simulink model "UserVehicle_RTW"  (Simulink 7.5)
settings: Solver=ode1  SolverMode=SingleTasking  StartTime=0.0  StopTime=inf  FixedStep=0.001  RelTol=1e-3
PreLoadFcn:
  | vehicle = 'Car'; if ~length(which('cmcmd')), cmenv; end
  | UserVehicle_RTW_bus
  | UserVehicle_RTW_params
InitFcn:
  | vehicle = 'Car'; if ~length(which('cmcmd')), cmenv; end
  | UserVehicle_RTW_bus
  | UserVehicle_RTW_params
values from neighbouring files (symbols this model uses):
  Car_Bdy1_mass = 650.0    (= 650)    [SingleTrack_RTW_params.m]    (also in UserVehicle_RTW_params.m)
  Car_Steering_i = 10.0    (= 10)    [SingleTrack_RTW_params.m]    (also in UserVehicle_RTW_params.m)
  Car_WhlBaseF = 1.5    [SingleTrack_RTW_params.m]    (also in UserVehicle_RTW_params.m)
  Car_WhlBaseR = -1.5    [SingleTrack_RTW_params.m]    (also in UserVehicle_RTW_params.m)
libraries: CarMaker4SL x77
(part 2 of 3)

== system UserVehicle_RTW/SingleTrack_Out/Subsystem1 ==
  In1 : Inport  OutDataType=sfix(16)  OutScaling=2^0
  Bus Creator : BusCreator  Inputs=3
  foo_Input_Selector1 : BusSelector  OutputSignals=Vhcl v,Vhcl Distance,Vhcl sRoad,Vhcl sRoadAero,Vhcl Hitch_Pos x,Vhcl Hitch_Pos y,Vhcl Hitch_Pos z,Vhcl Roll,Vhcl RollVel,Vhcl RollAcc,Vhcl Pitch,Vhcl PitchVel,Vhcl PitchAcc,Vhcl Yaw,Vhcl YawRate,Vhcl YawAcc
  Out1 : Outport  OutDataType=sfix(16)  OutScaling=2^0
  Out2 : Outport  Port=2  OutDataType=sfix(16)  OutScaling=2^0
  Out3 : Outport  Port=3  OutDataType=sfix(16)  OutScaling=2^0
  Out4 : Outport  Port=4  OutDataType=sfix(16)  OutScaling=2^0
  Out6 : Outport  Port=5  OutDataType=sfix(16)  OutScaling=2^0
  Out7 : Outport  Port=6  OutDataType=sfix(16)  OutScaling=2^0
  Out8 : Outport  Port=7  OutDataType=sfix(16)  OutScaling=2^0
  Out9 : Outport  Port=8  OutDataType=sfix(16)  OutScaling=2^0
  Out10 : Outport  Port=9  OutDataType=sfix(16)  OutScaling=2^0
  Out11 : Outport  Port=10  OutDataType=sfix(16)  OutScaling=2^0
  Out12 : Outport  Port=11  OutDataType=sfix(16)  OutScaling=2^0
  Out13 : Outport  Port=12  OutDataType=sfix(16)  OutScaling=2^0
  Out14 : Outport  Port=13  OutDataType=sfix(16)  OutScaling=2^0
  Out15 : Outport  Port=14  OutDataType=sfix(16)  OutScaling=2^0
  wires:
  In1/1 -> foo_Input_Selector1/1
  foo_Input_Selector1/16 -> Out15/1  "<Vhcl YawAcc>"
  foo_Input_Selector1/15 -> Out14/1  "<Vhcl YawRate>"
  foo_Input_Selector1/14 -> Out13/1  "<Vhcl Yaw>"
  foo_Input_Selector1/13 -> Out12/1  "<Vhcl PitchAcc>"
  foo_Input_Selector1/12 -> Out11/1  "<Vhcl PitchVel>"
  foo_Input_Selector1/11 -> Out10/1  "<Vhcl Pitch>"
  foo_Input_Selector1/10 -> Out9/1  "<Vhcl RollAcc>"
  foo_Input_Selector1/9 -> Out8/1  "<Vhcl RollVel>"
  foo_Input_Selector1/8 -> Out7/1  "<Vhcl Roll>"
  Bus Creator/1 -> Out6/1
  foo_Input_Selector1/4 -> Out4/1  "<Vhcl sRoadAero>"
  foo_Input_Selector1/3 -> Out3/1  "<Vhcl sRoad>"
  foo_Input_Selector1/2 -> Out2/1  "<Vhcl Distance>"
  foo_Input_Selector1/1 -> Out1/1  "<Vhcl v>"
  foo_Input_Selector1/7 -> Bus Creator/3  "<Vhcl Hitch_Pos z>"
  foo_Input_Selector1/6 -> Bus Creator/2  "<Vhcl Hitch_Pos y>"
  foo_Input_Selector1/5 -> Bus Creator/1  "<Vhcl Hitch_Pos x>"

== system UserVehicle_RTW/SingleTrack_Out/Subsystem2 ==
  In1 : Inport  OutDataType=sfix(16)  OutScaling=2^0
  Bus Creator : BusCreator  Inputs=3
  Bus Creator1 : BusCreator  Inputs=3
  foo_Input_Selector3 : BusSelector  OutputSignals=Vhcl Wheel FL t x,Vhcl Wheel FL t y,Vhcl Wheel FL t z,Vhcl Wheel FL r_zxy x,Vhcl Wheel FL r_zxy y,Vhcl Wheel FL r_zxy z,Vhcl Wheel FL Fx,Vhcl Wheel FL Fy,Vhcl Wheel FL Fz,Vhcl Wheel FL vBelt,Vhcl Wheel FL LongSlip,Vhcl Wheel FL SideSlip,Vhcl Wheel FL Trq_T2W,Vhcl Wheel FL Trq_WhlBearing
  Out1 : Outport  OutDataType=sfix(16)  OutScaling=2^0
  Out2 : Outport  Port=2  OutDataType=sfix(16)  OutScaling=2^0
  Out3 : Outport  Port=3  OutDataType=sfix(16)  OutScaling=2^0
  Out4 : Outport  Port=4  OutDataType=sfix(16)  OutScaling=2^0
  Out5 : Outport  Port=5  OutDataType=sfix(16)  OutScaling=2^0
  Out6 : Outport  Port=6  OutDataType=sfix(16)  OutScaling=2^0
  Out7 : Outport  Port=7  OutDataType=sfix(16)  OutScaling=2^0
  Out8 : Outport  Port=8  OutDataType=sfix(16)  OutScaling=2^0
  Out9 : Outport  Port=9  OutDataType=sfix(16)  OutScaling=2^0
  Out10 : Outport  Port=10  OutDataType=sfix(16)  OutScaling=2^0
  wires:
  foo_Input_Selector3/14 -> Out10/1  "<Vhcl Wheel FL Trq_WhlBearing>"
  foo_Input_Selector3/13 -> Out9/1  "<Vhcl Wheel FL Trq_T2W>"
  foo_Input_Selector3/12 -> Out8/1  "<Vhcl Wheel FL SideSlip>"
  foo_Input_Selector3/11 -> Out7/1  "<Vhcl Wheel FL LongSlip>"
  foo_Input_Selector3/10 -> Out6/1  "<Vhcl Wheel FL vBelt>"
  foo_Input_Selector3/9 -> Out5/1  "<Vhcl Wheel FL Fz>"
  foo_Input_Selector3/8 -> Out4/1  "<Vhcl Wheel FL Fy>"
  In1/1 -> foo_Input_Selector3/1
  foo_Input_Selector3/7 -> Out3/1  "<Vhcl Wheel FL Fx>"
  Bus Creator/1 -> Out2/1
  Bus Creator1/1 -> Out1/1
  foo_Input_Selector3/6 -> Bus Creator/3  "<Vhcl Wheel FL r_zxy z>"
  foo_Input_Selector3/5 -> Bus Creator/2  "<Vhcl Wheel FL r_zxy y>"
  foo_Input_Selector3/4 -> Bus Creator/1  "<Vhcl Wheel FL r_zxy x>"
  foo_Input_Selector3/3 -> Bus Creator1/3  "<Vhcl Wheel FL t z>"
  foo_Input_Selector3/2 -> Bus Creator1/2  "<Vhcl Wheel FL t y>"
  foo_Input_Selector3/1 -> Bus Creator1/1  "<Vhcl Wheel FL t x>"

== system UserVehicle_RTW/SingleTrack_Out/Subsystem3 ==
  In1 : Inport  OutDataType=sfix(16)  OutScaling=2^0
  Bus Creator : BusCreator  Inputs=3
  Bus Creator1 : BusCreator  Inputs=3
  foo_Input_Selector3 : BusSelector  OutputSignals=Vhcl Wheel FR t x,Vhcl Wheel FR t y,Vhcl Wheel FR t z,Vhcl Wheel FR r_zxy x,Vhcl Wheel FR r_zxy y,Vhcl Wheel FR r_zxy z,Vhcl Wheel FR Fx,Vhcl Wheel FR Fy,Vhcl Wheel FR Fz,Vhcl Wheel FR vBelt,Vhcl Wheel FR LongSlip,Vhcl Wheel FR SideSlip,Vhcl Wheel FR Trq_T2W,Vhcl Wheel FR Trq_WhlBearing
  Out1 : Outport  OutDataType=sfix(16)  OutScaling=2^0
  Out2 : Outport  Port=2  OutDataType=sfix(16)  OutScaling=2^0
  Out3 : Outport  Port=3  OutDataType=sfix(16)  OutScaling=2^0
  Out4 : Outport  Port=4  OutDataType=sfix(16)  OutScaling=2^0
  Out5 : Outport  Port=5  OutDataType=sfix(16)  OutScaling=2^0
  Out6 : Outport  Port=6  OutDataType=sfix(16)  OutScaling=2^0
  Out7 : Outport  Port=7  OutDataType=sfix(16)  OutScaling=2^0
  Out8 : Outport  Port=8  OutDataType=sfix(16)  OutScaling=2^0
  Out9 : Outport  Port=9  OutDataType=sfix(16)  OutScaling=2^0
  Out10 : Outport  Port=10  OutDataType=sfix(16)  OutScaling=2^0
  wires:
  foo_Input_Selector3/14 -> Out10/1  "<Vhcl Wheel FR Trq_WhlBearing>"
  foo_Input_Selector3/13 -> Out9/1  "<Vhcl Wheel FR Trq_T2W>"
  foo_Input_Selector3/12 -> Out8/1  "<Vhcl Wheel FR SideSlip>"
  foo_Input_Selector3/11 -> Out7/1  "<Vhcl Wheel FR LongSlip>"
  foo_Input_Selector3/10 -> Out6/1  "<Vhcl Wheel FR vBelt>"
  foo_Input_Selector3/9 -> Out5/1  "<Vhcl Wheel FR Fz>"
  foo_Input_Selector3/8 -> Out4/1  "<Vhcl Wheel FR Fy>"
  In1/1 -> foo_Input_Selector3/1
  foo_Input_Selector3/7 -> Out3/1  "<Vhcl Wheel FR Fx>"
  Bus Creator1/1 -> Out2/1
  Bus Creator/1 -> Out1/1
  foo_Input_Selector3/6 -> Bus Creator1/3  "<Vhcl Wheel FR r_zxy z>"
  foo_Input_Selector3/5 -> Bus Creator1/2  "<Vhcl Wheel FR r_zxy y>"
  foo_Input_Selector3/4 -> Bus Creator1/1  "<Vhcl Wheel FR r_zxy x>"
  foo_Input_Selector3/3 -> Bus Creator/3  "<Vhcl Wheel FR t z>"
  foo_Input_Selector3/2 -> Bus Creator/2  "<Vhcl Wheel FR t y>"
  foo_Input_Selector3/1 -> Bus Creator/1  "<Vhcl Wheel FR t x>"

== system UserVehicle_RTW/SingleTrack_Out/Subsystem4 ==
  In1 : Inport  OutDataType=sfix(16)  OutScaling=2^0
  Bus Creator : BusCreator  Inputs=3
  Bus Creator1 : BusCreator  Inputs=3
  foo_Input_Selector3 : BusSelector  OutputSignals=Vhcl Wheel RL t x,Vhcl Wheel RL t y,Vhcl Wheel RL t z,Vhcl Wheel RL r_zxy x,Vhcl Wheel RL r_zxy y,Vhcl Wheel RL r_zxy z,Vhcl Wheel RL Fx,Vhcl Wheel RL Fy,Vhcl Wheel RL Fz,Vhcl Wheel RL vBelt,Vhcl Wheel RL LongSlip,Vhcl Wheel RL SideSlip,Vhcl Wheel RL Trq_T2W,Vhcl Wheel RL Trq_WhlBearing
  Out1 : Outport  OutDataType=sfix(16)  OutScaling=2^0
  Out2 : Outport  Port=2  OutDataType=sfix(16)  OutScaling=2^0
  Out3 : Outport  Port=3  OutDataType=sfix(16)  OutScaling=2^0
  Out4 : Outport  Port=4  OutDataType=sfix(16)  OutScaling=2^0
  Out5 : Outport  Port=5  OutDataType=sfix(16)  OutScaling=2^0
  Out6 : Outport  Port=6  OutDataType=sfix(16)  OutScaling=2^0
  Out7 : Outport  Port=7  OutDataType=sfix(16)  OutScaling=2^0
  Out8 : Outport  Port=8  OutDataType=sfix(16)  OutScaling=2^0
  Out9 : Outport  Port=9  OutDataType=sfix(16)  OutScaling=2^0
  Out10 : Outport  Port=10  OutDataType=sfix(16)  OutScaling=2^0
  wires:
  foo_Input_Selector3/14 -> Out10/1  "<Vhcl Wheel RL Trq_WhlBearing>"
  foo_Input_Selector3/13 -> Out9/1  "<Vhcl Wheel RL Trq_T2W>"
  foo_Input_Selector3/12 -> Out8/1  "<Vhcl Wheel RL SideSlip>"
  foo_Input_Selector3/11 -> Out7/1  "<Vhcl Wheel RL LongSlip>"
  foo_Input_Selector3/10 -> Out6/1  "<Vhcl Wheel RL vBelt>"
  foo_Input_Selector3/9 -> Out5/1  "<Vhcl Wheel RL Fz>"
  foo_Input_Selector3/8 -> Out4/1  "<Vhcl Wheel RL Fy>"
  In1/1 -> foo_Input_Selector3/1
  foo_Input_Selector3/7 -> Out3/1  "<Vhcl Wheel RL Fx>"
  Bus Creator1/1 -> Out2/1
  Bus Creator/1 -> Out1/1
  foo_Input_Selector3/6 -> Bus Creator1/3  "<Vhcl Wheel RL r_zxy z>"
  foo_Input_Selector3/5 -> Bus Creator1/2  "<Vhcl Wheel RL r_zxy y>"
  foo_Input_Selector3/4 -> Bus Creator1/1  "<Vhcl Wheel RL r_zxy x>"
  foo_Input_Selector3/3 -> Bus Creator/3  "<Vhcl Wheel RL t z>"
  foo_Input_Selector3/2 -> Bus Creator/2  "<Vhcl Wheel RL t y>"
  foo_Input_Selector3/1 -> Bus Creator/1  "<Vhcl Wheel RL t x>"

== system UserVehicle_RTW/SingleTrack_Out/Subsystem5 ==
  In1 : Inport  OutDataType=sfix(16)  OutScaling=2^0
  Bus Creator : BusCreator  Inputs=3
  Bus Creator1 : BusCreator  Inputs=3
  foo_Input_Selector3 : BusSelector  OutputSignals=Vhcl Wheel RR t x,Vhcl Wheel RR t y,Vhcl Wheel RR t z,Vhcl Wheel RR r_zxy x,Vhcl Wheel RR r_zxy y,Vhcl Wheel RR r_zxy z,Vhcl Wheel RR Fx,Vhcl Wheel RR Fy,Vhcl Wheel RR Fz,Vhcl Wheel RR vBelt,Vhcl Wheel RR LongSlip,Vhcl Wheel RR SideSlip,Vhcl Wheel RR Trq_T2W,Vhcl Wheel RR Trq_WhlBearing
  Out1 : Outport  OutDataType=sfix(16)  OutScaling=2^0
  Out2 : Outport  Port=2  OutDataType=sfix(16)  OutScaling=2^0
  Out3 : Outport  Port=3  OutDataType=sfix(16)  OutScaling=2^0
  Out4 : Outport  Port=4  OutDataType=sfix(16)  OutScaling=2^0
  Out5 : Outport  Port=5  OutDataType=sfix(16)  OutScaling=2^0
  Out6 : Outport  Port=6  OutDataType=sfix(16)  OutScaling=2^0
  Out7 : Outport  Port=7  OutDataType=sfix(16)  OutScaling=2^0
  Out8 : Outport  Port=8  OutDataType=sfix(16)  OutScaling=2^0
  Out9 : Outport  Port=9  OutDataType=sfix(16)  OutScaling=2^0
  Out10 : Outport  Port=10  OutDataType=sfix(16)  OutScaling=2^0
  wires:
  foo_Input_Selector3/14 -> Out10/1  "<Vhcl Wheel RR Trq_WhlBearing>"
  foo_Input_Selector3/13 -> Out9/1  "<Vhcl Wheel RR Trq_T2W>"
  foo_Input_Selector3/12 -> Out8/1  "<Vhcl Wheel RR SideSlip>"
  foo_Input_Selector3/11 -> Out7/1  "<Vhcl Wheel RR LongSlip>"
  foo_Input_Selector3/10 -> Out6/1  "<Vhcl Wheel RR vBelt>"
  foo_Input_Selector3/9 -> Out5/1  "<Vhcl Wheel RR Fz>"
  foo_Input_Selector3/8 -> Out4/1  "<Vhcl Wheel RR Fy>"
  In1/1 -> foo_Input_Selector3/1
  foo_Input_Selector3/7 -> Out3/1  "<Vhcl Wheel RR Fx>"
  Bus Creator1/1 -> Out2/1
  Bus Creator/1 -> Out1/1
  foo_Input_Selector3/6 -> Bus Creator1/3  "<Vhcl Wheel RR r_zxy z>"
  foo_Input_Selector3/5 -> Bus Creator1/2  "<Vhcl Wheel RR r_zxy y>"
  foo_Input_Selector3/4 -> Bus Creator1/1  "<Vhcl Wheel RR r_zxy x>"
  foo_Input_Selector3/3 -> Bus Creator/3  "<Vhcl Wheel RR t z>"
  foo_Input_Selector3/2 -> Bus Creator/2  "<Vhcl Wheel RR t y>"
  foo_Input_Selector3/1 -> Bus Creator/1  "<Vhcl Wheel RR t x>"

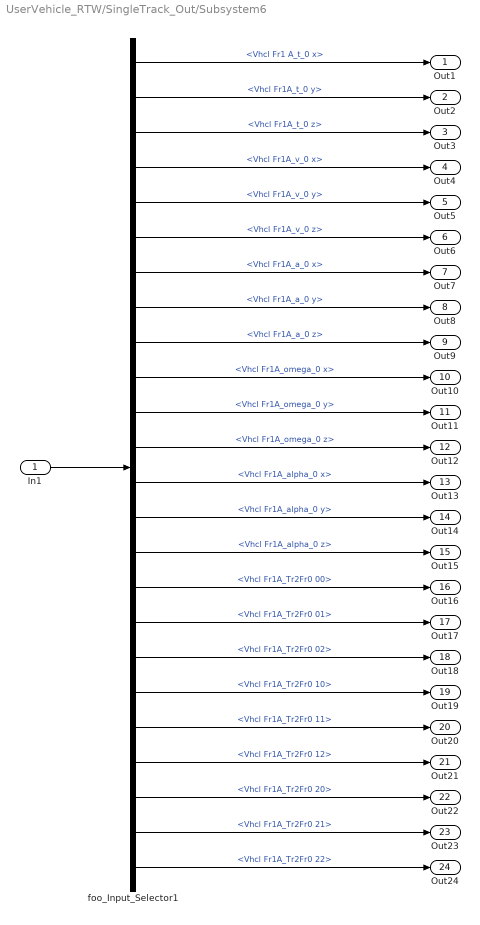
== system UserVehicle_RTW/SingleTrack_Out/Subsystem6 ==
  In1 : Inport  OutDataType=sfix(16)  OutScaling=2^0
  foo_Input_Selector1 : BusSelector  OutputSignals=Vhcl Fr1 A_t_0 x,Vhcl Fr1A_t_0 y,Vhcl Fr1A_t_0 z,Vhcl Fr1A_v_0 x,Vhcl Fr1A_v_0 y,Vhcl Fr1A_v_0 z,Vhcl Fr1A_a_0 x,Vhcl Fr1A_a_0 y,Vhcl Fr1A_a_0 z,Vhcl Fr1A_omega_0 x,Vhcl Fr1A_omega_0 y,Vhcl Fr1A_omega_0 z,Vhcl Fr1A_alpha_0 x,Vhcl Fr1A_alpha_0 y,Vhcl Fr1A_alpha_0 z,Vhcl Fr1A_Tr2Fr0 00,Vhcl Fr1A_Tr2Fr0 01,Vhcl Fr1A_Tr2Fr0 02,Vhcl Fr1A_Tr2Fr0 10,Vhcl Fr1A_Tr2Fr0 11,Vhcl Fr1A_Tr2Fr0 12,Vhcl Fr1A_Tr2Fr0 20,Vhcl Fr1A_Tr2Fr0 21,Vhcl Fr1A_Tr2Fr0 22
  Out1 : Outport  OutDataType=sfix(16)  OutScaling=2^0
  Out2 : Outport  Port=2  OutDataType=sfix(16)  OutScaling=2^0
  Out3 : Outport  Port=3  OutDataType=sfix(16)  OutScaling=2^0
  Out4 : Outport  Port=4  OutDataType=sfix(16)  OutScaling=2^0
  Out5 : Outport  Port=5  OutDataType=sfix(16)  OutScaling=2^0
  Out6 : Outport  Port=6  OutDataType=sfix(16)  OutScaling=2^0
  Out7 : Outport  Port=7  OutDataType=sfix(16)  OutScaling=2^0
  Out8 : Outport  Port=8  OutDataType=sfix(16)  OutScaling=2^0
  Out9 : Outport  Port=9  OutDataType=sfix(16)  OutScaling=2^0
  Out10 : Outport  Port=10  OutDataType=sfix(16)  OutScaling=2^0
  Out11 : Outport  Port=11  OutDataType=sfix(16)  OutScaling=2^0
  Out12 : Outport  Port=12  OutDataType=sfix(16)  OutScaling=2^0
  Out13 : Outport  Port=13  OutDataType=sfix(16)  OutScaling=2^0
  Out14 : Outport  Port=14  OutDataType=sfix(16)  OutScaling=2^0
  Out15 : Outport  Port=15  OutDataType=sfix(16)  OutScaling=2^0
  Out16 : Outport  Port=16  OutDataType=sfix(16)  OutScaling=2^0
  Out17 : Outport  Port=17  OutDataType=sfix(16)  OutScaling=2^0
  Out18 : Outport  Port=18  OutDataType=sfix(16)  OutScaling=2^0
  Out19 : Outport  Port=19  OutDataType=sfix(16)  OutScaling=2^0
  Out20 : Outport  Port=20  OutDataType=sfix(16)  OutScaling=2^0
  Out21 : Outport  Port=21  OutDataType=sfix(16)  OutScaling=2^0
  Out22 : Outport  Port=22  OutDataType=sfix(16)  OutScaling=2^0
  Out23 : Outport  Port=23  OutDataType=sfix(16)  OutScaling=2^0
  Out24 : Outport  Port=24  OutDataType=sfix(16)  OutScaling=2^0
  wires:
  foo_Input_Selector1/15 -> Out15/1  "<Vhcl Fr1A_alpha_0 z>"
  foo_Input_Selector1/14 -> Out14/1  "<Vhcl Fr1A_alpha_0 y>"
  foo_Input_Selector1/13 -> Out13/1  "<Vhcl Fr1A_alpha_0 x>"
  foo_Input_Selector1/12 -> Out12/1  "<Vhcl Fr1A_omega_0 z>"
  foo_Input_Selector1/11 -> Out11/1  "<Vhcl Fr1A_omega_0 y>"
  foo_Input_Selector1/10 -> Out10/1  "<Vhcl Fr1A_omega_0 x>"
  foo_Input_Selector1/9 -> Out9/1  "<Vhcl Fr1A_a_0 z>"
  foo_Input_Selector1/8 -> Out8/1  "<Vhcl Fr1A_a_0 y>"
  foo_Input_Selector1/7 -> Out7/1  "<Vhcl Fr1A_a_0 x>"
  foo_Input_Selector1/6 -> Out6/1  "<Vhcl Fr1A_v_0 z>"
  foo_Input_Selector1/5 -> Out5/1  "<Vhcl Fr1A_v_0 y>"
  foo_Input_Selector1/4 -> Out4/1  "<Vhcl Fr1A_v_0 x>"
  foo_Input_Selector1/3 -> Out3/1  "<Vhcl Fr1A_t_0 z>"
  foo_Input_Selector1/2 -> Out2/1  "<Vhcl Fr1A_t_0 y>"
  foo_Input_Selector1/1 -> Out1/1  "<Vhcl Fr1 A_t_0 x>"
  In1/1 -> foo_Input_Selector1/1
  foo_Input_Selector1/16 -> Out16/1  "<Vhcl Fr1A_Tr2Fr0 00>"
  foo_Input_Selector1/17 -> Out17/1  "<Vhcl Fr1A_Tr2Fr0 01>"
  foo_Input_Selector1/18 -> Out18/1  "<Vhcl Fr1A_Tr2Fr0 02>"
  foo_Input_Selector1/19 -> Out19/1  "<Vhcl Fr1A_Tr2Fr0 10>"
  foo_Input_Selector1/20 -> Out20/1  "<Vhcl Fr1A_Tr2Fr0 11>"
  foo_Input_Selector1/21 -> Out21/1  "<Vhcl Fr1A_Tr2Fr0 12>"
  foo_Input_Selector1/22 -> Out22/1  "<Vhcl Fr1A_Tr2Fr0 20>"
  foo_Input_Selector1/23 -> Out23/1  "<Vhcl Fr1A_Tr2Fr0 21>"
  foo_Input_Selector1/24 -> Out24/1  "<Vhcl Fr1A_Tr2Fr0 22>"

== system UserVehicle_RTW/UserVehicle/CreateBus Car.Hitch.FrcTrq ==
  Bus Creator : BusCreator  Inputs=6
  Constant{1..2,7..10} (6 alike) : Constant  Value=0
  Demux7 : Demux  Outputs=6
  Mux1 : Mux  Inputs=6
  Car.Hitch.FrcTrq : Outport
  wires:
  Constant1/1 -> Mux1/6
  Constant2/1 -> Mux1/5
  Constant7/1 -> Mux1/1
  Constant10/1 -> Mux1/4
  Constant9/1 -> Mux1/3
  Constant8/1 -> Mux1/2
  Mux1/1 -> Demux7/1
  Bus Creator/1 -> Car.Hitch.FrcTrq/1
  Demux7/6 -> Bus Creator/6  "Car Hitch Trq2Car z"
  Demux7/5 -> Bus Creator/5  "Car Hitch Trq2Car y"
  Demux7/4 -> Bus Creator/4  "Car Hitch Trq2Car x"
  Demux7/3 -> Bus Creator/3  "Car Hitch Frc2Car z"
  Demux7/2 -> Bus Creator/2  "Car Hitch Frc2Car y"
  Demux7/1 -> Bus Creator/1  "Car Hitch Frc2Car x"

== system UserVehicle_RTW/UserVehicle/CreateBus Vhcl.Fr1 ==
  Vhcl.Fr1_In : Inport
  BdyFrame2Vhcl.Fr1A : Subsystem
  Ground : Ground
  Ground1 : Ground
  Tr2Fr0 : Subsystem
  a_0 : Subsystem
  t_0 : Subsystem
  v_0 : Subsystem
  Vhcl.Fr1A : Outport
  wires:
  Ground/1 -> BdyFrame2Vhcl.Fr1A/5(alpha_0)
  Ground1/1 -> BdyFrame2Vhcl.Fr1A/4(omega_0)
  a_0/1(a_0) -> BdyFrame2Vhcl.Fr1A/3(a_0)
  v_0/1(v_0) -> BdyFrame2Vhcl.Fr1A/2(v_0)
  t_0/1(t_0) -> BdyFrame2Vhcl.Fr1A/1(t_0)
  Tr2Fr0/1(Tr2Fr0) -> BdyFrame2Vhcl.Fr1A/6(Tr2Fr0), a_0/2(Tr2Fr0), v_0/2(Tr2Fr0)
  Vhcl.Fr1_In/1 -> Tr2Fr0/1(Car), t_0/1(Car), v_0/1(Car), a_0/1(Car)
  BdyFrame2Vhcl.Fr1A/1(Vhcl.Fr1) -> Vhcl.Fr1A/1

== system UserVehicle_RTW/UserVehicle/CreateBus Vhcl.Misc ==
  In1 : Inport
  Bus Creator5 : BusCreator  Inputs=11
  Demux5 : Demux  Outputs=11
  Out1 : Outport
  wires:
  Demux5/11 -> Bus Creator5/11  "Vhcl Wind_vel_0 z"
  Demux5/10 -> Bus Creator5/10  "Vhcl Wind_vel_0 y"
  Demux5/9 -> Bus Creator5/9  "Vhcl Wind_vel_0 x"
  Demux5/8 -> Bus Creator5/8  "Vhcl DL2BdyEng y"
  Demux5/7 -> Bus Creator5/7  "Vhcl DL2BdyEng x"
  Demux5/6 -> Bus Creator5/6  "Vhcl TrqDL2Bdy1B z"
  Demux5/5 -> Bus Creator5/5  "Vhcl TrqDL2Bdy1B y"
  Demux5/4 -> Bus Creator5/4  "Vhcl TrqDL2Bdy1B x"
  Demux5/3 -> Bus Creator5/3  "Vhcl Trq_DL2Bdy1 z"
  In1/1 -> Demux5/1
  Bus Creator5/1 -> Out1/1
  Demux5/2 -> Bus Creator5/2  "Vhcl Trq_DL2Bdy1 y"
  Demux5/1 -> Bus Creator5/1  "Vhcl Trq_DL2Bdy1 x"

== system UserVehicle_RTW/UserVehicle/CreateBus Vhcl.Motion ==
  Vhcl_Motion_In : Inport
  Bus Creator : BusCreator  Inputs=16
  Bus Selector : BusSelector  OutputSignals=Car_v_1.Car_vx_1,Car_Dist,Car_sRoad,Road_Fr1_rx,Road_Fr1_ry,Car_Yaw.Yaw,Car_Yaw.Yawp,Car_Yaw.Yawpp
  Constant{2..4,6..7,9..10} (7 alike) : Constant  Value=0
  Demux1 : Demux  Outputs=16
  Mux1 : Mux  Inputs=16
  Vhcl.Motion : Outport
  wires:
  Bus Selector/3 -> Mux1/3, Mux1/4  "<Car_sRoad>"
  Bus Selector/5 -> Mux1/11  "<Road_Fr1_ry>"
  Bus Selector/4 -> Mux1/8  "<Road_Fr1_rx>"
  Bus Selector/8 -> Mux1/16  "<Yawpp>"
  Bus Selector/7 -> Mux1/15  "<Yawp>"
  Bus Selector/6 -> Mux1/14  "<Yaw>"
  Constant10/1 -> Mux1/13
  Constant9/1 -> Mux1/12
  Constant7/1 -> Mux1/10
  Constant6/1 -> Mux1/9
  Constant4/1 -> Mux1/7
  Constant3/1 -> Mux1/6
  Constant2/1 -> Mux1/5
  Bus Selector/2 -> Mux1/2  "<Car_Dist>"
  Bus Selector/1 -> Mux1/1  "<Car_vx_1>"
  Mux1/1 -> Demux1/1
  Bus Creator/1 -> Vhcl.Motion/1
  Demux1/1 -> Bus Creator/1  "Vhcl v"
  Demux1/2 -> Bus Creator/2  "Vhcl Distance"
  Demux1/3 -> Bus Creator/3  "Vhcl sRoad"
  Demux1/4 -> Bus Creator/4  "Vhcl sRoadAero"
  Demux1/5 -> Bus Creator/5  "Vhcl Hitch_Pos x"
  Demux1/6 -> Bus Creator/6  "Vhcl Hitch_Pos y"
  Demux1/7 -> Bus Creator/7  "Vhcl Hitch_Pos z"
  Demux1/8 -> Bus Creator/8  "Vhcl Roll"
  Demux1/9 -> Bus Creator/9  "Vhcl RollVel"
  Demux1/10 -> Bus Creator/10  "Vhcl RollAcc"
  Demux1/11 -> Bus Creator/11  "Vhcl Pitch"
  Demux1/12 -> Bus Creator/12  "Vhcl PitchVel"
  Demux1/13 -> Bus Creator/13  "Vhcl PitchAcc"
  Demux1/14 -> Bus Creator/14  "Vhcl Yaw"
  Demux1/15 -> Bus Creator/15  "Vhcl YawRate"
  Demux1/16 -> Bus Creator/16  "Vhcl YawAcc"
  Vhcl_Motion_In/1 -> Bus Selector/1

== system UserVehicle_RTW/UserVehicle/CreateBus Vhcl.PT ==
  In1 : Inport
  Bus Creator3 : BusCreator  Inputs=6
  Demux3 : Demux  Outputs=6
  Out1 : Outport
  wires:
  In1/1 -> Demux3/1
  Bus Creator3/1 -> Out1/1
  Demux3/4 -> Bus Creator3/4  "VhclCtrl SelectorCtrl"
  Demux3/2 -> Bus Creator3/2  "VhclCtrl SST"
  Demux3/1 -> Bus Creator3/1  "VhclCtrl Key"
  Demux3/5 -> Bus Creator3/5  "VhclCtrl SelectorManualShift"
  Demux3/3 -> Bus Creator3/3  "VhclCtrl StarterCtrl"
  Demux3/6 -> Bus Creator3/6  "VhclCtrl Gas"

== system UserVehicle_RTW/UserVehicle/CreateBus Vhcl.PoI ==
  Vhcl_POI_In : Inport
  Bus Creator : BusCreator  Inputs=18
  Bus Selector : BusSelector  OutputSignals=Car_t_0.Car_tx_0,Car_t_0.Car_ty_0,Road_Fr1_z,Car_v_0.Car_vx_0,Car_v_0.Car_vy_0,Car_a_0.Car_ax_0,Car_a_0.Car_ay_0,Car_v_1.Car_vx_1,Car_v_1.Car_vy_1,Car_a_1.Car_ax_1,Car_a_1.Car_ay_1
  Constant{11..13,15..16,18..19} (7 alike) : Constant  Value=0
  Demux3 : Demux  Outputs=18
  Mux1 : Mux  Inputs=18
  Vhcl.PoI : Outport
  wires:
  Bus Selector/8 -> Mux1/10  "<Car_vx_1>"
  Bus Selector/7 -> Mux1/8  "<Car_ay_0>"
  Constant19/1 -> Mux1/15
  Bus Selector/11 -> Mux1/14  "<Car_ay_1>"
  Bus Selector/10 -> Mux1/13  "<Car_ax_1>"
  Constant18/1 -> Mux1/12
  Constant16/1 -> Mux1/9
  Bus Selector/6 -> Mux1/7  "<Car_ax_0>"
  Constant15/1 -> Mux1/6
  Bus Selector/5 -> Mux1/5  "<Car_vy_0>"
  Bus Selector/4 -> Mux1/4  "<Car_vx_0>"
  Bus Selector/3 -> Mux1/3  "<Road_Fr1_z>"
  Bus Selector/2 -> Mux1/2  "<Car_ty_0>"
  Bus Selector/1 -> Mux1/1  "<Car_tx_0>"
  Constant11/1 -> Mux1/18
  Constant13/1 -> Mux1/17
  Constant12/1 -> Mux1/16
  Vhcl_POI_In/1 -> Bus Selector/1
  Mux1/1 -> Demux3/1
  Demux3/18 -> Bus Creator/18  "Vhcl PoI_GCS Elev"
  Demux3/17 -> Bus Creator/17  "Vhcl PoI_GCS Lat"
  Demux3/16 -> Bus Creator/16  "Vhcl PoI_GCS Long"
  Demux3/15 -> Bus Creator/15  "Vhcl PoI_Acc_1 z"
  Demux3/14 -> Bus Creator/14  "Vhcl PoI_Acc_1 y"
  Demux3/13 -> Bus Creator/13  "Vhcl PoI_Acc_1 x"
  Demux3/12 -> Bus Creator/12  "Vhcl PoI_Vel_1 z"
  Demux3/11 -> Bus Creator/11  "Vhcl PoI_Vel_1 y"
  Demux3/10 -> Bus Creator/10  "Vhcl PoI_Vel_1 x"
  Demux3/9 -> Bus Creator/9  "Vhcl PoI_Acc z"
  Demux3/8 -> Bus Creator/8  "Vhcl PoI_Acc y"
  Demux3/7 -> Bus Creator/7  "Vhcl PoI_Acc x"
  Demux3/6 -> Bus Creator/6  "Vhcl PoI_Vel z"
  Demux3/5 -> Bus Creator/5  "Vhcl PoI_Vel y"
  Demux3/4 -> Bus Creator/4  "Vhcl PoI_Vel x"
  Demux3/3 -> Bus Creator/3  "Vhcl PoI_Pos z"
  Demux3/2 -> Bus Creator/2  "Vhcl PoI_Pos y"
  Bus Creator/1 -> Vhcl.PoI/1
  Demux3/1 -> Bus Creator/1  "Vhcl PoI_Pos x"
  Bus Selector/9 -> Mux1/11  "<Car_vy_1>"

== system UserVehicle_RTW/UserVehicle/CreateBus Vhcl.Steering ==
  Vhcl_Steering_In : Inport
  Bus Creator : BusCreator
  Bus Selector : BusSelector  OutputSignals=VhclCtrl Steering Ang,VhclCtrl Steering AngVel,VhclCtrl Steering AngAcc,VhclCtrl Steering Trq
  Demux : Demux
  Mux1 : Mux
  Vhcl.Steering : Outport
  wires:
  Mux1/1 -> Demux/1
  Bus Selector/4 -> Mux1/4  "<VhclCtrl Steering Trq>"
  Bus Selector/3 -> Mux1/3  "<VhclCtrl Steering AngAcc>"
  Bus Selector/2 -> Mux1/2  "<VhclCtrl Steering AngVel>"
  Bus Selector/1 -> Mux1/1  "<VhclCtrl Steering Ang>"
  Vhcl_Steering_In/1 -> Bus Selector/1
  Bus Creator/1 -> Vhcl.Steering/1
  Demux/1 -> Bus Creator/1  "Vhcl Steering Ang"
  Demux/3 -> Bus Creator/3  "Vhcl Steering AngAcc"
  Demux/2 -> Bus Creator/2  "Vhcl Steering AngVel"
  Demux/4 -> Bus Creator/4  "Vhcl Steering Trq"

== system UserVehicle_RTW/UserVehicle/CreateBus Vhcl.Wheel.FL ==
  Vhcl.Wheel.FL_In : Inport
  Bus Creator : BusCreator  Inputs=14
  Bus Selector : BusSelector  OutputSignals=Car_Whl_F_rz,Car_Tire.Car_Tire_F.LongFrc,Car_Tire.Car_Tire_F.SideFrc,Car_Whl_F_1.Car_F_Fz_1,Car_Tire.Car_Tire_F.vBelt,Car_Tire.Car_Tire_F.Slp,Car_Tire.Car_Tire_F.Alpha,Car_Trq2W.Trq_F
  Constant{1..5,11} (6 alike) : Constant  Value=0
  Demux3 : Demux  Outputs=14
  Mux1 : Mux  Inputs=14
  Vhcl.Wheel.FL : Outport
  wires:
  Bus Selector/4 -> Mux1/9  "<Car_F_Fz_1>"
  Constant11/1 -> Mux1/14
  Bus Selector/8 -> Mux1/13  "<Trq_F>"
  Bus Selector/6 -> Mux1/11  "<Slp>"
  Bus Selector/3 -> Mux1/8  "<SideFrc>"
  Bus Selector/2 -> Mux1/7  "<LongFrc>"
  Constant5/1 -> Mux1/5
  Constant4/1 -> Mux1/4
  Constant3/1 -> Mux1/3
  Constant2/1 -> Mux1/2
  Constant1/1 -> Mux1/1
  Bus Selector/1 -> Mux1/6  "<Car_Whl_F_rz>"
  Vhcl.Wheel.FL_In/1 -> Bus Selector/1
  Demux3/14 -> Bus Creator/14  "Vhcl Wheel FL Trq_WhlBearing"
  Demux3/13 -> Bus Creator/13  "Vhcl Wheel FL Trq_T2W"
  Demux3/12 -> Bus Creator/12  "Vhcl Wheel FL SideSlip"
  Demux3/11 -> Bus Creator/11  "Vhcl Wheel FL LongSlip"
  Demux3/10 -> Bus Creator/10  "Vhcl Wheel FL vBelt"
  Demux3/9 -> Bus Creator/9  "Vhcl Wheel FL Fz"
  Demux3/8 -> Bus Creator/8  "Vhcl Wheel FL Fy"
  Demux3/7 -> Bus Creator/7  "Vhcl Wheel FL Fx"
  Demux3/6 -> Bus Creator/6  "Vhcl Wheel FL r_zxy z"
  Demux3/5 -> Bus Creator/5  "Vhcl Wheel FL r_zxy y"
  Demux3/4 -> Bus Creator/4  "Vhcl Wheel FL r_zxy x"
  Demux3/3 -> Bus Creator/3  "Vhcl Wheel FL t z"
  Demux3/2 -> Bus Creator/2  "Vhcl Wheel FL t y"
  Mux1/1 -> Demux3/1
  Bus Creator/1 -> Vhcl.Wheel.FL/1
  Demux3/1 -> Bus Creator/1  "Vhcl Wheel FL t x"
  Bus Selector/5 -> Mux1/10  "<vBelt>"
  Bus Selector/7 -> Mux1/12  "<Alpha>"

== system UserVehicle_RTW/UserVehicle/CreateBus Vhcl.Wheel.FR ==
  Vhcl.Wheel.FR_In : Inport
  Bus Creator : BusCreator  Inputs=14
  Bus Selector : BusSelector  OutputSignals=Car_Whl_F_rz,Car_Tire.Car_Tire_F.LongFrc,Car_Tire.Car_Tire_F.SideFrc,Car_Whl_F_1.Car_F_Fz_1,Car_Tire.Car_Tire_F.vBelt,Car_Tire.Car_Tire_F.Slp,Car_Tire.Car_Tire_F.Alpha,Car_Trq2W.Trq_F
  Constant{1..5,11} (6 alike) : Constant  Value=0
  Demux3 : Demux  Outputs=14
  Mux1 : Mux  Inputs=14
  Vhcl.Wheel.FR : Outport
  wires:
  Constant11/1 -> Mux1/14
  Bus Selector/8 -> Mux1/13  "<Trq_F>"
  Bus Selector/6 -> Mux1/11  "<Slp>"
  Bus Selector/5 -> Mux1/10  "<vBelt>"
  Bus Selector/7 -> Mux1/12  "<Alpha>"
  Bus Selector/4 -> Mux1/9  "<Car_F_Fz_1>"
  Bus Selector/3 -> Mux1/8  "<SideFrc>"
  Bus Selector/2 -> Mux1/7  "<LongFrc>"
  Constant5/1 -> Mux1/5
  Constant4/1 -> Mux1/4
  Constant3/1 -> Mux1/3
  Constant2/1 -> Mux1/2
  Constant1/1 -> Mux1/1
  Bus Selector/1 -> Mux1/6  "<Car_Whl_F_rz>"
  Vhcl.Wheel.FR_In/1 -> Bus Selector/1
  Mux1/1 -> Demux3/1
  Demux3/14 -> Bus Creator/14  "Vhcl Wheel FR Trq_WhlBearing"
  Demux3/13 -> Bus Creator/13  "Vhcl Wheel FR Trq_T2W"
  Demux3/12 -> Bus Creator/12  "Vhcl Wheel FR SideSlip"
  Demux3/11 -> Bus Creator/11  "Vhcl Wheel FR LongSlip"
  Demux3/10 -> Bus Creator/10  "Vhcl Wheel FR vBelt"
  Demux3/9 -> Bus Creator/9  "Vhcl Wheel FR Fz"
  Demux3/8 -> Bus Creator/8  "Vhcl Wheel FR Fy"
  Demux3/7 -> Bus Creator/7  "Vhcl Wheel FR Fx"
  Demux3/6 -> Bus Creator/6  "Vhcl Wheel FR r_zxy z"
  Demux3/5 -> Bus Creator/5  "Vhcl Wheel FR r_zxy y"
  Demux3/4 -> Bus Creator/4  "Vhcl Wheel FR r_zxy x"
  Demux3/3 -> Bus Creator/3  "Vhcl Wheel FR t z"
  Demux3/2 -> Bus Creator/2  "Vhcl Wheel FR t y"
  Bus Creator/1 -> Vhcl.Wheel.FR/1
  Demux3/1 -> Bus Creator/1  "Vhcl Wheel FR t x"

== system UserVehicle_RTW/UserVehicle/CreateBus Vhcl.Wheel.In ==
  In1 : Inport
  Bus Creator1 : BusCreator  Inputs=12
  Demux1 : Demux  Outputs=12
  Out1 : Outport
  wires:
  Demux1/12 -> Bus Creator1/12  "Vhcl Wheel RR rotv"
  Demux1/11 -> Bus Creator1/11  "Vhcl Wheel RR Trq_DL2WC"
  Demux1/10 -> Bus Creator1/10  "Vhcl Wheel RR Trq_B2WC"
  Demux1/9 -> Bus Creator1/9  "Vhcl Wheel RL rotv"
  Demux1/8 -> Bus Creator1/8  "Vhcl Wheel RL Trq_DL2WC"
  Demux1/7 -> Bus Creator1/7  "Vhcl Wheel RL Trq_B2WC"
  Demux1/6 -> Bus Creator1/6  "Vhcl Wheel FR rotv"
  Demux1/5 -> Bus Creator1/5  "Vhcl Wheel FR Trq_DL2WC"
  Demux1/4 -> Bus Creator1/4  "Vhcl Wheel FR Trq_B2WC"
  Demux1/3 -> Bus Creator1/3  "Vhcl Wheel FL rotv"
  In1/1 -> Demux1/1
  Bus Creator1/1 -> Out1/1
  Demux1/2 -> Bus Creator1/2  "Vhcl Wheel FL Trq_DL2WC"
  Demux1/1 -> Bus Creator1/1  "Vhcl Wheel FL Trq_B2WC"

== system UserVehicle_RTW/UserVehicle/CreateBus Vhcl.Wheel.RL ==
  Vhcl.Wheel.RL_In : Inport
  Bus Creator : BusCreator  Inputs=14
  Bus Selector : BusSelector  OutputSignals=Car_Tire.Car_Tire_R.LongFrc,Car_Tire.Car_Tire_R.SideFrc,Car_Whl_F_1.Car_R_Fz_1,Car_Tire.Car_Tire_R.Alpha,Car_Trq2W.Trq_R
  Constant{1..5,9..11,13} (9 alike) : Constant  Value=0
  Demux3 : Demux  Outputs=14
  Mux1 : Mux  Inputs=14
  Vhcl.Wheel.RL : Outport
  wires:
  Bus Selector/4 -> Mux1/12  "<Alpha>"
  Constant13/1 -> Mux1/6
  Constant11/1 -> Mux1/14
  Bus Selector/5 -> Mux1/13  "<Trq_R>"
  Constant10/1 -> Mux1/11
  Constant9/1 -> Mux1/10
  Bus Selector/3 -> Mux1/9  "<Car_R_Fz_1>"
  Bus Selector/2 -> Mux1/8  "<SideFrc>"
  Bus Selector/1 -> Mux1/7  "<LongFrc>"
  Constant5/1 -> Mux1/5
  Constant4/1 -> Mux1/4
  Constant3/1 -> Mux1/3
  Constant2/1 -> Mux1/2
  Constant1/1 -> Mux1/1
  Vhcl.Wheel.RL_In/1 -> Bus Selector/1
  Mux1/1 -> Demux3/1
  Demux3/14 -> Bus Creator/14  "Vhcl Wheel RL Trq_WhlBearing"
  Demux3/13 -> Bus Creator/13  "Vhcl Wheel RL Trq_T2W"
  Demux3/12 -> Bus Creator/12  "Vhcl Wheel RL SideSlip"
  Demux3/11 -> Bus Creator/11  "Vhcl Wheel RL LongSlip"
  Demux3/10 -> Bus Creator/10  "Vhcl Wheel RL vBelt"
  Demux3/9 -> Bus Creator/9  "Vhcl Wheel RL Fz"
  Demux3/8 -> Bus Creator/8  "Vhcl Wheel RL Fy"
  Demux3/7 -> Bus Creator/7  "Vhcl Wheel RL Fx"
  Demux3/6 -> Bus Creator/6  "Vhcl Wheel RL r_zxy z"
  Demux3/5 -> Bus Creator/5  "Vhcl Wheel RL r_zxy y"
  Demux3/4 -> Bus Creator/4  "Vhcl Wheel RL r_zxy x"
  Demux3/3 -> Bus Creator/3  "Vhcl Wheel RL t z"
  Demux3/2 -> Bus Creator/2  "Vhcl Wheel RL t y"
  Bus Creator/1 -> Vhcl.Wheel.RL/1
  Demux3/1 -> Bus Creator/1  "Vhcl Wheel RL t x"

== system UserVehicle_RTW/UserVehicle/CreateBus Vhcl.Wheel.RR ==
  Vhcl.Wheel.RR_In : Inport
  Bus Creator : BusCreator  Inputs=14
  Bus Selector : BusSelector  OutputSignals=Car_Tire.Car_Tire_R.LongFrc,Car_Tire.Car_Tire_R.SideFrc,Car_Whl_F_1.Car_R_Fz_1,Car_Tire.Car_Tire_R.Alpha,Car_Trq2W.Trq_R
  Constant{1..5,9..11,13} (9 alike) : Constant  Value=0
  Demux3 : Demux  Outputs=14
  Mux1 : Mux  Inputs=14
  Vhcl.Wheel.RR : Outport
  wires:
  Bus Selector/4 -> Mux1/12  "<Alpha>"
  Constant13/1 -> Mux1/6
  Constant11/1 -> Mux1/14
  Bus Selector/5 -> Mux1/13  "<Trq_R>"
  Constant10/1 -> Mux1/11
  Constant9/1 -> Mux1/10
  Bus Selector/3 -> Mux1/9  "<Car_R_Fz_1>"
  Bus Selector/2 -> Mux1/8  "<SideFrc>"
  Constant5/1 -> Mux1/5
  Constant4/1 -> Mux1/4
  Constant3/1 -> Mux1/3
  Constant2/1 -> Mux1/2
  Constant1/1 -> Mux1/1
  Vhcl.Wheel.RR_In/1 -> Bus Selector/1
  Mux1/1 -> Demux3/1
  Demux3/14 -> Bus Creator/14  "Vhcl Wheel RR Trq_WhlBearing"
  Demux3/13 -> Bus Creator/13  "Vhcl Wheel RR Trq_T2W"
  Demux3/12 -> Bus Creator/12  "Vhcl Wheel RR SideSlip"
  Demux3/11 -> Bus Creator/11  "Vhcl Wheel RR LongSlip"
  Demux3/10 -> Bus Creator/10  "Vhcl Wheel RR vBelt"
  Demux3/9 -> Bus Creator/9  "Vhcl Wheel RR Fz"
  Demux3/8 -> Bus Creator/8  "Vhcl Wheel RR Fy"
  Demux3/7 -> Bus Creator/7  "Vhcl Wheel RR Fx"
  Demux3/6 -> Bus Creator/6  "Vhcl Wheel RR r_zxy z"
  Demux3/5 -> Bus Creator/5  "Vhcl Wheel RR r_zxy y"
  Demux3/4 -> Bus Creator/4  "Vhcl Wheel RR r_zxy x"
  Demux3/3 -> Bus Creator/3  "Vhcl Wheel RR t z"
  Demux3/2 -> Bus Creator/2  "Vhcl Wheel RR t y"
  Demux3/1 -> Bus Creator/1  "Vhcl Wheel RR t x"
  Bus Selector/1 -> Mux1/7  "<LongFrc>"
  Bus Creator/1 -> Vhcl.Wheel.RR/1

== system UserVehicle_RTW/UserVehicle/CreateBus VhclCtrl.Steering ==
  In1 : Inport
  Bus Creator : BusCreator  Inputs=5
  Demux : Demux  Outputs=5
  Out1 : Outport
  wires:
  In1/1 -> Demux/1
  Bus Creator/1 -> Out1/1
  Demux/1 -> Bus Creator/1  "VhclCtrl Steering Ang"
  Demux/5 -> Bus Creator/5  "VhclCtrl Steering ByTrq"
  Demux/3 -> Bus Creator/3  "VhclCtrl Steering AngAcc"
  Demux/2 -> Bus Creator/2  "VhclCtrl Steering AngVel"
  Demux/4 -> Bus Creator/4  "VhclCtrl Steering Trq"

== system UserVehicle_RTW/UserVehicle/Query Road CoG ==
  In1 : Inport
  Bus Selector1 : BusSelector  OutputSignals=Car_t_0.Car_tx_0,Car_t_0.Car_ty_0,Car_Dist
  Bus Selector2 : BusSelector  OutputSignals=z,slope,grade,s
  Constant1 : Constant  Value=0
  Constant2 : Constant  Value=0
  Mux : Mux  Inputs=3
  Read CM Parameter : CarMaker4SL/Read CM Parameter  xfile=Vehicle  xkey=Wheel.fl.pos  xnout=1  xdefaults=0  xmuxed=on
  Subsystem : Subsystem
  Sum2 : Sum  SaturateOnIntegerOverflow=on  InputSameDT=on  OutDataTypeStr=Inherit: Same as first input
  neg : Gain  Gain=-1  SaturateOnIntegerOverflow=on  OutDataTypeStr=Inherit: Same as input  ParamDataTypeStr=Inherit: Same as input
  Fr1_z : Outport
  Fr1_rx : Outport  Port=2
  Fr1_ry : Outport  Port=3
  sRoad : Outport  Port=4
  wires:
  Read CM Parameter/1 -> Sum2/2
  Sum2/1 -> sRoad/1
  Bus Selector2/4 -> Sum2/1  "<s>"
  neg/1 -> Fr1_ry/1
  Bus Selector2/3 -> neg/1  "<grade>"
  Constant1/1 -> Subsystem/3(Side)
  Subsystem/1(Tire) -> Bus Selector2/1
  Bus Selector1/1 -> Mux/1  "<Car_tx_0>"
  Bus Selector1/2 -> Mux/2  "<Car_ty_0>"
  Mux/1 -> Subsystem/1(xyz)
  Bus Selector1/3 -> Subsystem/2(Dist)  "<Car_Dist>"
  In1/1 -> Bus Selector1/1
  Bus Selector2/1 -> Fr1_z/1  "<z>"
  Bus Selector2/2 -> Fr1_rx/1  "<slope>"
  Constant2/1 -> Mux/3
  [TRSim] -> Subsystem/Enable

== system UserVehicle_RTW/UserVehicle/SimStates ==
  note: Detect CarMaker states and transistions relevant for initialization at the start of a new testrun.
  Logical Operator : Logic  AllPortsSameDT=off  OutDataTypeMode=boolean  OutDataTypeStr=boolean
  Logical Operator1 : Logic  Operator=OR  AllPortsSameDT=off  OutDataTypeMode=boolean  OutDataTypeStr=boolean
  Memory : Memory
  Read CM Dict : CarMaker4SL/Read CM Dict  xname=SC.State  xsync=off
  Read CM Dict1 : CarMaker4SL/Read CM Dict  xname=Time  xsync=off
  Relational Operator : RelationalOperator  Operator=<=  LogicOutDataTypeMode=boolean  OutDataTypeStr=boolean
  Relational Operator1 : RelationalOperator  Operator===  LogicOutDataTypeMode=boolean  OutDataTypeStr=boolean
  Relational Operator2 : RelationalOperator  Operator===  LogicOutDataTypeMode=boolean  OutDataTypeStr=boolean
  SCState_Simulate : Constant  Value=8
  Zero : Constant  Value=0
  detect increase : RelationalOperator  Operator=>  LogicOutDataTypeMode=boolean  OutDataTypeStr=boolean
  tag scope: TRSim=global, TRStart=global
  wires:
  Memory/1 -> detect increase/2
  detect increase/1 -> Logical Operator/1
  Logical Operator1/1 -> [TRStart]
  Logical Operator/1 -> Logical Operator1/2
  Relational Operator2/1 -> Logical Operator1/1
  Zero/1 -> Relational Operator2/2
  Read CM Dict1/1 -> Relational Operator2/1
  Relational Operator1/1 -> [TRSim]
  Relational Operator/1 -> Logical Operator/2
  SCState_Simulate/1 -> Relational Operator1/1, Relational Operator/2
  Read CM Dict/1 -> detect increase/1, Memory/1, Relational Operator1/2, Relational Operator/1

== system UserVehicle_RTW/UserVehicle/Single Track Model ==
  note: Formeln nach:
      | Schramm, Hiller, Bardini
      | Modellbildung und Simulation der Dynamik von Kraftfahrzeugen
      | Seite 244 ff
      | ISBN 978-3-540-89313-4
  VhclCtrl.Steering : Inport
  Vhcl.Wheel.In : Inport  Port=2
  Tire2Wheel : Subsystem
  sideslip angle : Subsystem
  steer kinematic : Subsystem
  tire forces : Subsystem
  vehicle motion : Subsystem
  wheel torques : Subsystem
  yaw : Subsystem
  Car.a_1 : Outport
  Car.v_1 : Outport  Port=2
  Car.a_0 : Outport  Port=3
  Car.v_0 : Outport  Port=4
  Car.t_0 : Outport  Port=5
  Car.Dist : Outport  Port=6
  Car.Yaw : Outport  Port=7
  Car.Tire : Outport  Port=8
  Car.Trq2W : Outport  Port=9
  Car.Whl.F.rz : Outport  Port=10
  Car.Whl.F_1 : Outport  Port=11
  wires:
  yaw/1(Car.Yaw) -> Car.Yaw/1, tire forces/1(Yaw), sideslip angle/3(Yaw), vehicle motion/3(Car_Yaw)
  wheel torques/1(Car.Trq2W) -> Car.Trq2W/1
  VhclCtrl.Steering/1 -> steer kinematic/1(In1)
  steer kinematic/1(Car.Whl.F.rz) -> Car.Whl.F.rz/1, tire forces/6(Car.Wheel.rz), Tire2Wheel/2(Wheel_rz)
  vehicle motion/2(Car.v_1) -> tire forces/3(Car_v_1), Car.v_1/1, sideslip angle/2(Car_v_1)
  sideslip angle/1(beta) -> tire forces/2(beta), vehicle motion/2(Car.Beta)  "beta"
  vehicle motion/1(Car.a_1) -> Car.a_1/1, sideslip angle/1(Car_a_1)
  vehicle motion/6(Car.Dist) -> Car.Dist/1
  vehicle motion/3(Car.a_0) -> Car.a_0/1
  vehicle motion/4(Car.v_0) -> Car.v_0/1
  vehicle motion/5(Car_t_0) -> Car.t_0/1, tire forces/4(Car_t_0)
  Vhcl.Wheel.In/1 -> tire forces/5(Vhcl.Wheel.In)
  tire forces/1(Tire) -> Tire2Wheel/1(Tire), Car.Tire/1, wheel torques/1(WheelTrq_1)
  Tire2Wheel/1(Car.Whl.F_1) -> yaw/1(WheelFrc_1), Car.Whl.F_1/1, tire forces/7(Car.Whl.F_1), vehicle motion/1(Car.Whl.F_1)

== system UserVehicle_RTW/UserVehicle/CreateBus Vhcl.Fr1/BdyFrame2Vhcl.Fr1A ==
  note: Translate pseudo BdyFrame interface to Vhcl.Fr1
  t_0 : Inport
  v_0 : Inport  Port=2
  a_0 : Inport  Port=3
  omega_0 : Inport  Port=4
  alpha_0 : Inport  Port=5
  Tr2Fr0 : Inport  Port=6
  Bus Creator : BusCreator  Inputs=24
  Demux{,1..3,5} (5 alike) : Demux  Outputs=3
  Demux4 : Demux  Outputs=9
  Vhcl.Fr1 : Outport
  wires:
  t_0/1 -> Demux/1
  v_0/1 -> Demux1/1
  a_0/1 -> Demux2/1
  omega_0/1 -> Demux3/1
  alpha_0/1 -> Demux5/1
  Tr2Fr0/1 -> Demux4/1
  Demux4/9 -> Bus Creator/24  "Vhcl Fr1A_Tr2Fr0 22"
  Demux4/8 -> Bus Creator/23  "Vhcl Fr1A_Tr2Fr0 21"
  Demux4/7 -> Bus Creator/22  "Vhcl Fr1A_Tr2Fr0 20"
  Demux4/6 -> Bus Creator/21  "Vhcl Fr1A_Tr2Fr0 12"
  Demux4/5 -> Bus Creator/20  "Vhcl Fr1A_Tr2Fr0 11"
  Demux4/4 -> Bus Creator/19  "Vhcl Fr1A_Tr2Fr0 10"
  Demux4/3 -> Bus Creator/18  "Vhcl Fr1A_Tr2Fr0 02"
  Demux4/2 -> Bus Creator/17  "Vhcl Fr1A_Tr2Fr0 01"
  Demux4/1 -> Bus Creator/16  "Vhcl Fr1A_Tr2Fr0 00"
  Demux5/3 -> Bus Creator/15  "Vhcl Fr1A_alpha_0 z"
  Demux5/2 -> Bus Creator/14  "Vhcl Fr1A_alpha_0 y"
  Demux5/1 -> Bus Creator/13  "Vhcl Fr1A_alpha_0 x"
  Demux3/3 -> Bus Creator/12  "Vhcl Fr1A_omega_0 z"
  Demux3/2 -> Bus Creator/11  "Vhcl Fr1A_omega_0 y"
  Demux3/1 -> Bus Creator/10  "Vhcl Fr1A_omega_0 x"
  Demux2/3 -> Bus Creator/9  "Vhcl Fr1A_a_0 z"
  Demux2/2 -> Bus Creator/8  "Vhcl Fr1A_a_0 y"
  Demux2/1 -> Bus Creator/7  "Vhcl Fr1A_a_0 x"
  Demux1/3 -> Bus Creator/6  "Vhcl Fr1A_v_0 z"
  Demux1/2 -> Bus Creator/5  "Vhcl Fr1A_v_0 y"
  Demux1/1 -> Bus Creator/4  "Vhcl Fr1A_v_0 x"
  Demux/3 -> Bus Creator/3  "Vhcl Fr1A_t_0 z"
  Demux/2 -> Bus Creator/2  "Vhcl Fr1A_t_0 y"
  Demux/1 -> Bus Creator/1  "Vhcl Fr1 A_t_0 x"
  Bus Creator/1 -> Vhcl.Fr1/1

== system UserVehicle_RTW/UserVehicle/CreateBus Vhcl.Fr1/Tr2Fr0 ==
  Car : Inport
  Bus Creator : BusCreator  Inputs=9
  Subsystem_00 : Subsystem
  Subsystem_01 : Subsystem
  Subsystem_02 : Subsystem
  Subsystem_10 : Subsystem
  Subsystem_11 : Subsystem
  Subsystem_12 : Subsystem
  Subsystem_20 : Subsystem
  Subsystem_21 : Subsystem
  Subsystem_22 : Subsystem
  sincos : Subsystem
  Tr2Fr0 : Outport
  wires:
  Car/1 -> sincos/1(Car)
  sincos/1(sincos) -> Subsystem_10/1(sincos), Subsystem_11/1(sincos), Subsystem_20/1(sincos), Subsystem_21/1(sincos), Subsystem_22/1(sincos), Subsystem_12/1(sincos), Subsystem_00/1(sincos), Subsystem_01/1(sincos), Subsystem_02/1(sincos)
  Bus Creator/1 -> Tr2Fr0/1
  Subsystem_00/1(Tr2Fr1_00) -> Bus Creator/1  "Tr2Fr0_00"
  Subsystem_10/1(Tr2Fr1_10) -> Bus Creator/4  "Tr2Fr0_10"
  Subsystem_20/1(Tr2Fr1_20) -> Bus Creator/7  "Tr2Fr0_20"
  Subsystem_21/1(Tr2Fr1_21) -> Bus Creator/8  "Tr2Fr0_21"
  Subsystem_22/1(Tr2Fr1_22) -> Bus Creator/9  "Tr2Fr0_22"
  Subsystem_01/1(Tr2Fr1_01) -> Bus Creator/2  "Tr2Fr0_01"
  Subsystem_02/1(Tr2Fr1_02) -> Bus Creator/3  "Tr2Fr0_02"
  Subsystem_11/1(Tr2Fr1_11) -> Bus Creator/5  "Tr2Fr1_11"
  Subsystem_12/1(Tr2Fr1_12) -> Bus Creator/6  "Tr2Fr1_12"

== system UserVehicle_RTW/UserVehicle/CreateBus Vhcl.Fr1/a_0 ==
  Car : Inport
  Tr2Fr0 : Inport  Port=2
  Add : Sum
  Add1 : Sum
  Add2 : Sum
  Bus Selector1 : BusSelector  OutputSignals=Car_a_1.Car_ax_1,Car_a_1.Car_ay_1
  Bus Selector2 : BusSelector  OutputSignals=Tr2Fr0_00,Tr2Fr0_01,Tr2Fr0_10,Tr2Fr1_11,Tr2Fr0_20,Tr2Fr0_21
  Mux1 : Mux  Inputs=3
  Product{,1..5} (6 alike) : Product  RndMeth=Zero
  a_0 : Outport
  wires:
  Mux1/1 -> a_0/1
  Car/1 -> Bus Selector1/1
  Tr2Fr0/1 -> Bus Selector2/1
  Bus Selector1/2 -> Product/1, Product2/1, Product4/1  "<Car_ay_1>"
  Bus Selector1/1 -> Product1/1, Product3/1, Product5/1  "<Car_ax_1>"
  Product1/1 -> Add/1
  Product/1 -> Add/2
  Add/1 -> Mux1/1
  Product3/1 -> Add1/1
  Product2/1 -> Add1/2
  Bus Selector2/1 -> Product1/2  "<Tr2Fr0_00>"
  Bus Selector2/2 -> Product/2  "<Tr2Fr0_01>"
  Add1/1 -> Mux1/2
  Bus Selector2/3 -> Product3/2  "<Tr2Fr0_10>"
  Bus Selector2/4 -> Product2/2  "<Tr2Fr1_11>"
  Product5/1 -> Add2/1
  Product4/1 -> Add2/2
  Add2/1 -> Mux1/3
  Bus Selector2/6 -> Product4/2  "<Tr2Fr0_21>"
  Bus Selector2/5 -> Product5/2  "<Tr2Fr0_20>"

== system UserVehicle_RTW/UserVehicle/CreateBus Vhcl.Fr1/t_0 ==
  Car : Inport
  Bus Selector : BusSelector  OutputSignals=Car_t_0.Car_tx_0,Car_t_0.Car_ty_0,Road_Fr1_z
  Mux : Mux  Inputs=3
  t_0 : Outport
  wires:
  Bus Selector/1 -> Mux/1  "<Car_tx_0>"
  Bus Selector/2 -> Mux/2  "<Car_ty_0>"
  Bus Selector/3 -> Mux/3  "<Road_Fr1_z>"
  Car/1 -> Bus Selector/1
  Mux/1 -> t_0/1

== system UserVehicle_RTW/UserVehicle/CreateBus Vhcl.Fr1/v_0 ==
  Car : Inport
  Tr2Fr0 : Inport  Port=2
  Bus Selector1 : BusSelector  OutputSignals=Car_v_1.Car_vx_1
  Bus Selector2 : BusSelector  OutputSignals=Tr2Fr0_00,Tr2Fr0_10,Tr2Fr0_20
  Mux1 : Mux  Inputs=3
  Product : Product  RndMeth=Zero
  Product1 : Product  RndMeth=Zero
  Product2 : Product  RndMeth=Zero
  v_0 : Outport
  wires:
  Car/1 -> Bus Selector1/1
  Mux1/1 -> v_0/1
  Tr2Fr0/1 -> Bus Selector2/1
  Bus Selector2/1 -> Product/2  "<Tr2Fr0_00>"
  Bus Selector2/2 -> Product1/2  "<Tr2Fr0_10>"
  Bus Selector2/3 -> Product2/2  "<Tr2Fr0_20>"
  Bus Selector1/1 -> Product/1, Product1/1, Product2/1  "<Car_vx_1>"
  Product/1 -> Mux1/1
  Product1/1 -> Mux1/2
  Product2/1 -> Mux1/3

== system UserVehicle_RTW/UserVehicle/Query Road CoG/Subsystem ==
  xyz : Inport
  Dist : Inport  Port=2
  Side : Inport  Port=3
  Enable : EnablePort
  IPGRoad5 : CarMaker4SL/IPGRoad5  SystemSampleTime=-1  xname=IPGRoad  xevalmode=RouteEval XY_S  xconsiderbumps=off  xusepath=off  xwithcurve=off  xabort=on
  Mux : Mux  Inputs=2
  Terminator : Terminator
  Tire : Outport
  wires:
  IPGRoad5/2 -> Tire/1
  xyz/1 -> IPGRoad5/2
  Mux/1 -> IPGRoad5/1
  Side/1 -> Mux/2
  Dist/1 -> Mux/1
  IPGRoad5/1 -> Terminator/1

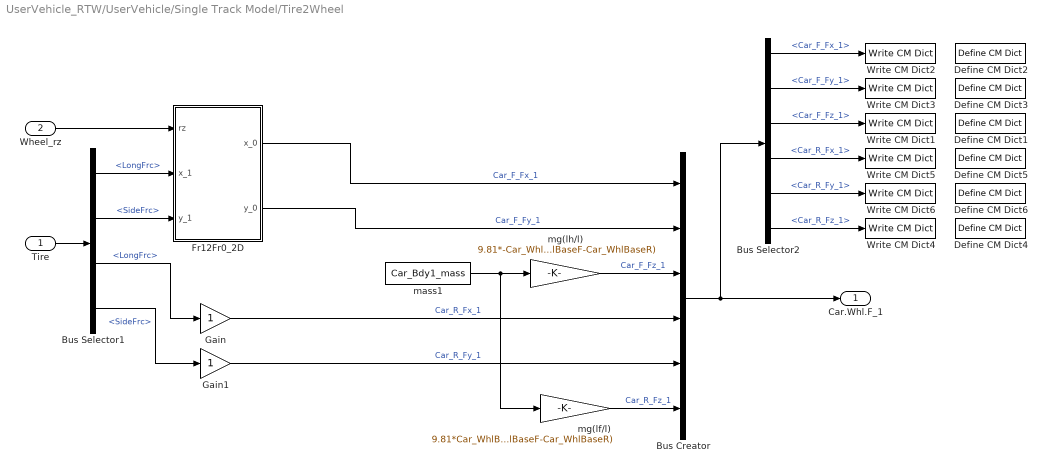
== system UserVehicle_RTW/UserVehicle/Single Track Model/Tire2Wheel ==
  Tire : Inport
  Wheel_rz : Inport  Port=2
  Bus Creator : BusCreator  Inputs=6
  Bus Selector1 : BusSelector  OutputSignals=Car_Tire_F.LongFrc,Car_Tire_F.SideFrc,Car_Tire_R.LongFrc,Car_Tire_R.SideFrc
  Bus Selector2 : BusSelector  OutputSignals=Car_F_Fx_1,Car_F_Fy_1,Car_F_Fz_1,Car_R_Fx_1,Car_R_Fy_1,Car_R_Fz_1
  Define CM Dict1 : CarMaker4SL/Define CM Dict  xname=Car.F.Fz_1  xunit=N  xmono=off  xtype=Double4  xdvaplace=None  xnstates=0  xfirststate=0  xinitial=0
  Define CM Dict2 : CarMaker4SL/Define CM Dict  xname=Car.F.Fx_1  xunit=N  xmono=off  xtype=Double4  xdvaplace=None  xnstates=0  xfirststate=0  xinitial=0
  Define CM Dict3 : CarMaker4SL/Define CM Dict  xname=Car.F.Fy_1  xunit=N  xmono=off  xtype=Double4  xdvaplace=None  xnstates=0  xfirststate=0  xinitial=0
  Define CM Dict4 : CarMaker4SL/Define CM Dict  xname=Car.R.Fz_1  xunit=N  xmono=off  xtype=Double4  xdvaplace=None  xnstates=0  xfirststate=0  xinitial=0
  Define CM Dict5 : CarMaker4SL/Define CM Dict  xname=Car.R.Fx_1  xunit=N  xmono=off  xtype=Double4  xdvaplace=None  xnstates=0  xfirststate=0  xinitial=0
  Define CM Dict6 : CarMaker4SL/Define CM Dict  xname=Car.R.Fy_1  xunit=N  xmono=off  xtype=Double4  xdvaplace=None  xnstates=0  xfirststate=0  xinitial=0
  Fr12Fr0_2D : Subsystem
  Gain : Gain
  Gain1 : Gain
  Write CM Dict1 : CarMaker4SL/Write CM Dict  xname=Car.F.Fz_1  xsync=off
  Write CM Dict2 : CarMaker4SL/Write CM Dict  xname=Car.F.Fx_1  xsync=off
  Write CM Dict3 : CarMaker4SL/Write CM Dict  xname=Car.F.Fy_1  xsync=off
  Write CM Dict4 : CarMaker4SL/Write CM Dict  xname=Car.R.Fz_1  xsync=off
  Write CM Dict5 : CarMaker4SL/Write CM Dict  xname=Car.R.Fx_1  xsync=off
  Write CM Dict6 : CarMaker4SL/Write CM Dict  xname=Car.R.Fy_1  xsync=off
  mass1 : Constant  Value=Car_Bdy1_mass
  mg(lf/l) : Gain  Gain=9.81*Car_WhlBaseF/(Car_WhlBaseF-Car_WhlBaseR)  SaturateOnIntegerOverflow=on  OutDataTypeStr=Inherit: Same as input  ParamDataTypeStr=Inherit: Same as input
  mg(lh/l) : Gain  Gain=9.81*-Car_WhlBaseR/(Car_WhlBaseF-Car_WhlBaseR)  SaturateOnIntegerOverflow=on  OutDataTypeStr=Inherit: Same as input  ParamDataTypeStr=Inherit: Same as input
  Car.Whl.F_1 : Outport
  wires:
  Tire/1 -> Bus Selector1/1
  Bus Creator/1 -> Car.Whl.F_1/1, Bus Selector2/1
  Bus Selector1/1 -> Fr12Fr0_2D/2(x_1)  "<LongFrc>"
  Bus Selector1/2 -> Fr12Fr0_2D/3(y_1)  "<SideFrc>"
  Bus Selector1/3 -> Gain/1  "<LongFrc>"
  Bus Selector1/4 -> Gain1/1  "<SideFrc>"
  Gain/1 -> Bus Creator/4  "Car_R_Fx_1"
  Gain1/1 -> Bus Creator/5  "Car_R_Fy_1"
  Fr12Fr0_2D/2(y_0) -> Bus Creator/2  "Car_F_Fy_1"
  Wheel_rz/1 -> Fr12Fr0_2D/1(rz)
  mass1/1 -> mg(lh/l)/1, mg(lf/l)/1
  mg(lh/l)/1 -> Bus Creator/3  "Car_F_Fz_1"
  mg(lf/l)/1 -> Bus Creator/6  "Car_R_Fz_1"
  Bus Selector2/1 -> Write CM Dict2/1  "<Car_F_Fx_1>"
  Bus Selector2/2 -> Write CM Dict3/1  "<Car_F_Fy_1>"
  Bus Selector2/3 -> Write CM Dict1/1  "<Car_F_Fz_1>"
  Bus Selector2/4 -> Write CM Dict5/1  "<Car_R_Fx_1>"
  Bus Selector2/5 -> Write CM Dict6/1  "<Car_R_Fy_1>"
  Bus Selector2/6 -> Write CM Dict4/1  "<Car_R_Fz_1>"
  Fr12Fr0_2D/1(x_0) -> Bus Creator/1  "Car_F_Fx_1"

== system UserVehicle_RTW/UserVehicle/Single Track Model/sideslip angle ==
  Car_a_1 : Inport
  Car_v_1 : Inport  Port=2
  Yaw : Inport  Port=3
  "  " : Product  SaturateOnIntegerOverflow=on  InputSameDT=on  OutDataTypeStr=Inherit: Same as first input
  Bus Creator : BusCreator  Inputs=2
  Bus Selector1 : BusSelector  OutputSignals=Yawp
  Bus Selector2 : BusSelector  OutputSignals=Car_ay_1,Car_ax_1
  Bus Selector3 : BusSelector  OutputSignals=Car_vx_1
  Define CM Dict : CarMaker4SL/Define CM Dict  xname=Car.SideSlipAngVel  xunit=rad/s  xmono=off  xtype=Double4  xdvaplace=None  xnstates=0  xfirststate=0  xinitial=0
  Define CM Dict1 : CarMaker4SL/Define CM Dict  xname=Car.SideSlipAng  xunit=rad  xmono=off  xtype=Double4  xdvaplace=None  xnstates=0  xfirststate=0  xinitial=0
  Subsystem : Subsystem
  Sum2 : Sum  Inputs=+-  SaturateOnIntegerOverflow=on  InputSameDT=on  OutDataTypeStr=Inherit: Same as first input
  Write CM Dict : CarMaker4SL/Write CM Dict  xname=Car.SideSlipAngVel  xsync=off
  Write CM Dict1 : CarMaker4SL/Write CM Dict  xname=Car.SideSlipAng  xsync=off
  beta_dot * dt : Integrator  ExternalReset=level
  beta : Outport
  wires:
  [TRStart] -> beta_dot * dt/2
  "  "/1 -> Sum2/2
  Sum2/1 -> Subsystem/3(In3)
  Car_v_1/1 -> Bus Selector3/1
  Yaw/1 -> Bus Selector1/1
  Bus Selector1/1 -> Subsystem/1(vYaw)  "<Yawp>"
  Bus Creator/1 -> beta/1
  Car_a_1/1 -> Bus Selector2/1
  Bus Selector2/1 -> Sum2/1  "<Car_ay_1>"
  Bus Selector2/2 -> "  "/1  "<Car_ax_1>"
  Bus Selector3/1 -> Subsystem/2(v)  "<Car_vx_1>"
  beta_dot * dt/1 -> Bus Creator/1, Write CM Dict1/1, "  "/2  "beta"
  Subsystem/1(Out1) -> beta_dot * dt/1, Bus Creator/2, Write CM Dict/1  "betap"

== system UserVehicle_RTW/UserVehicle/Single Track Model/steer kinematic ==
  In1 : Inport
  Bus Selector4 : BusSelector  OutputSignals=VhclCtrl Steering Ang
  "Steering_i " : Gain  Gain=1/Car_Steering_i  SaturateOnIntegerOverflow=on  OutDataTypeStr=Inherit: Same as input  ParamDataTypeStr=Inherit: Same as input
  Car.Whl.F.rz : Outport
  wires:
  Bus Selector4/1 -> "Steering_i "/1  "<VhclCtrl Steering Ang>"
  In1/1 -> Bus Selector4/1
  "Steering_i "/1 -> Car.Whl.F.rz/1
